simulink model "CognitiveOperator"  (R2017a)
settings: Solver=VariableStepAuto  StartTime=0.0  StopTime=81  RelTol=1e-3
values from neighbouring files (symbols this model uses):
  b = 0.1    [DCMotVal.mat]
  J = 0.01    [DCMotVal.mat]
  K = 0.01    [DCMotVal.mat]
  L = 0.5    [DCMotVal.mat]
  R = 1    [DCMotVal.mat]
libraries: simulink x1
settings Model: PauseTimes=1  Creator=Igor Khimchenko  LastModifiedBy=Igor Khimchenko

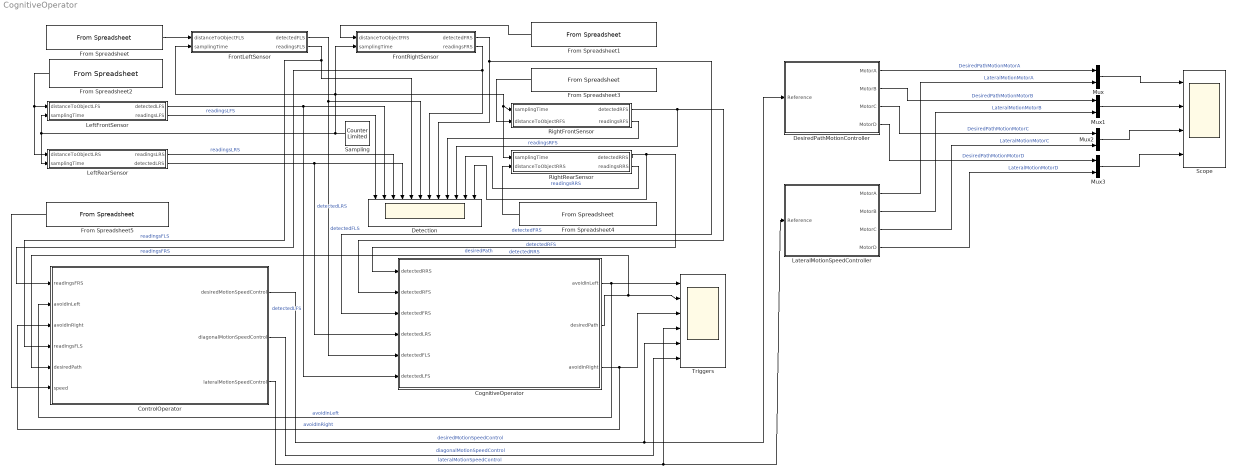
== system CognitiveOperator ==
  CognitiveOperator : Stateflow chart  TreatAsAtomicUnit=on
  ControlOperator : Stateflow chart  TreatAsAtomicUnit=on
  DesiredPathMotionController : Subsystem
  Detection : Scope  NumInputPorts=12
  From Spreadsheet : FromSpreadsheet  FileName=SensorReadings.xlsx  SheetName=Front left
  From Spreadsheet1 : FromSpreadsheet  FileName=SensorReadings.xlsx  SheetName=Front right
  From Spreadsheet2 : FromSpreadsheet  FileName=SensorReadings.xlsx  SheetName=Left
  From Spreadsheet3 : FromSpreadsheet  FileName=SensorReadings.xlsx  SheetName=Right front
  From Spreadsheet4 : FromSpreadsheet  FileName=SensorReadings.xlsx  SheetName=Right rear
  From Spreadsheet5 : FromSpreadsheet  FileName=SensorReadings.xlsx  SheetName=Speed
  FrontLeftSensor : Stateflow chart  TreatAsAtomicUnit=on
  FrontRightSensor : Stateflow chart  TreatAsAtomicUnit=on
  LateralMotionSpeedController : Subsystem
  LeftFrontSensor : Stateflow chart  TreatAsAtomicUnit=on
  LeftRearSensor : Stateflow chart  TreatAsAtomicUnit=on
  Mux{,1..3} (4 alike) : Mux  Inputs=2
  RightFrontSensor : Stateflow chart  TreatAsAtomicUnit=on
  RightRearSensor : Stateflow chart  TreatAsAtomicUnit=on
  Sampling : simulink/Sources/Counter Limited  uplimit=50  tsamp=0.001
  Scope : Scope  NumInputPorts=4
  Triggers : Scope  NumInputPorts=6
  wires:
  From Spreadsheet2/1 -> LeftRearSensor/1(distanceToObjectLRS), LeftFrontSensor/1(distanceToObjectLFS)
  Sampling/1 -> LeftRearSensor/2(samplingTime), LeftFrontSensor/2(samplingTime), FrontRightSensor/2(samplingTime), RightRearSensor/1(samplingTime), RightFrontSensor/1(samplingTime), FrontLeftSensor/2(samplingTime)
  LeftFrontSensor/2(readingsLFS) -> Detection/1  "readingsLFS"
  LeftFrontSensor/1(detectedLFS) -> CognitiveOperator/6(detectedLFS), Detection/2  "detectedLFS"
  LeftRearSensor/1(readingsLRS) -> Detection/3  "readingsLRS"
  LeftRearSensor/2(detectedLRS) -> CognitiveOperator/4(detectedLRS), Detection/4  "detectedLRS"
  FrontLeftSensor/2(readingsFLS) -> ControlOperator/4(readingsFLS), Detection/5  "readingsFLS"
  FrontLeftSensor/1(detectedFLS) -> CognitiveOperator/5(detectedFLS), Detection/6  "detectedFLS"
  FrontRightSensor/2(readingsFRS) -> ControlOperator/1(readingsFRS), Detection/7  "readingsFRS"
  FrontRightSensor/1(detectedFRS) -> CognitiveOperator/3(detectedFRS), Detection/8  "detectedFRS"
  RightFrontSensor/2(readingsRFS) -> Detection/9  "readingsRFS"
  RightFrontSensor/1(detectedRFS) -> Detection/10, CognitiveOperator/2(detectedRFS)  "detectedRFS"
  RightRearSensor/2(readingsRRS) -> Detection/11  "readingsRRS"
  RightRearSensor/1(detectedRRS) -> CognitiveOperator/1(detectedRRS), Detection/12  "detectedRRS"
  CognitiveOperator/1(avoidInLeft) -> ControlOperator/2(avoidInLeft), Triggers/1  "avoidInLeft"
  CognitiveOperator/2(desiredPath) -> ControlOperator/5(desiredPath), Triggers/2  "desiredPath"
  CognitiveOperator/3(avoidInRight) -> ControlOperator/3(avoidInRight), Triggers/3  "avoidInRight"
  From Spreadsheet3/1 -> RightFrontSensor/2(distanceToObjectRFS)
  From Spreadsheet4/1 -> RightRearSensor/2(distanceToObjectRRS)
  ControlOperator/1(desiredMotionSpeedControl) -> Triggers/5, DesiredPathMotionController/1(Reference)  "desiredMotionSpeedControl"
  ControlOperator/3(lateralMotionSpeedControl) -> Triggers/4, LateralMotionSpeedController/1(Reference)  "lateralMotionSpeedControl"
  From Spreadsheet5/1 -> ControlOperator/6(speed)
  From Spreadsheet/1 -> FrontLeftSensor/1(distanceToObjectFLS)
  From Spreadsheet1/1 -> FrontRightSensor/1(distanceToObjectFRS)
  ControlOperator/2(diagonalMotionSpeedControl) -> Triggers/6  "diagonalMotionSpeedControl"
  Mux/1 -> Scope/1
  Mux1/1 -> Scope/2
  Mux2/1 -> Scope/3
  Mux3/1 -> Scope/4
  DesiredPathMotionController/1(MotorA) -> Mux/1  "DesiredPathMotionMotorA"
  DesiredPathMotionController/2(MotorB) -> Mux1/1  "DesiredPathMotionMotorB"
  DesiredPathMotionController/3(MotorC) -> Mux2/1  "DesiredPathMotionMotorC"
  DesiredPathMotionController/4(MotorD) -> Mux3/1  "DesiredPathMotionMotorD"
  LateralMotionSpeedController/1(MotorA) -> Mux/2  "LateralMotionMotorA"
  LateralMotionSpeedController/2(MotorB) -> Mux1/2  "LateralMotionMotorB"
  LateralMotionSpeedController/3(MotorC) -> Mux2/2  "LateralMotionMotorC"
  LateralMotionSpeedController/4(MotorD) -> Mux3/2  "LateralMotionMotorD"

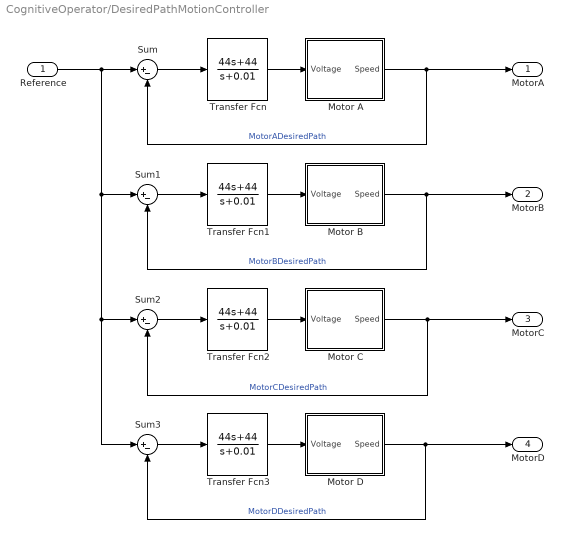
== system CognitiveOperator/DesiredPathMotionController ==
  Reference : Inport
  Motor A : Subsystem
  Motor B : Subsystem
  Motor C : Subsystem
  Motor D : Subsystem
  Sum{,1..3} (4 alike) : Sum  Inputs=|+-
  Transfer Fcn{,1..3} (4 alike) : TransferFcn  Numerator=[44 44]  Denominator=[1 0.01]
  MotorA : Outport
  MotorB : Outport  Port=2
  MotorC : Outport  Port=3
  MotorD : Outport  Port=4
  wires:
  Transfer Fcn/1 -> Motor A/1(Voltage)
  Sum2/1 -> Transfer Fcn2/1
  Transfer Fcn1/1 -> Motor B/1(Voltage)
  Sum1/1 -> Transfer Fcn1/1
  Motor D/1(Speed) -> MotorD/1, Sum3/2  "MotorDDesiredPath"
  Sum3/1 -> Transfer Fcn3/1
  Motor A/1(Speed) -> MotorA/1, Sum/2  "MotorADesiredPath"
  Motor C/1(Speed) -> MotorC/1, Sum2/2  "MotorCDesiredPath"
  Sum/1 -> Transfer Fcn/1
  Transfer Fcn3/1 -> Motor D/1(Voltage)
  Reference/1 -> Sum3/1, Sum2/1, Sum1/1, Sum/1
  Motor B/1(Speed) -> MotorB/1, Sum1/2  "MotorBDesiredPath"
  Transfer Fcn2/1 -> Motor C/1(Voltage)

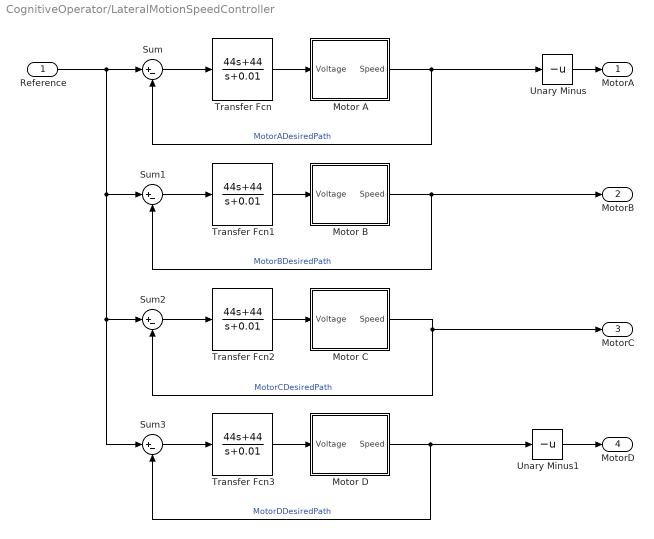
== system CognitiveOperator/LateralMotionSpeedController ==
  Reference : Inport
  Motor A : Subsystem
  Motor B : Subsystem
  Motor C : Subsystem
  Motor D : Subsystem
  Sum{,1..3} (4 alike) : Sum  Inputs=|+-
  Transfer Fcn{,1..3} (4 alike) : TransferFcn  Numerator=[44 44]  Denominator=[1 0.01]
  Unary Minus : UnaryMinus
  Unary Minus1 : UnaryMinus
  MotorA : Outport
  MotorB : Outport  Port=2
  MotorC : Outport  Port=3
  MotorD : Outport  Port=4
  wires:
  Sum/1 -> Transfer Fcn/1
  Transfer Fcn/1 -> Motor A/1(Voltage)
  Sum2/1 -> Transfer Fcn2/1
  Sum3/1 -> Transfer Fcn3/1
  Motor C/1(Speed) -> MotorC/1, Sum2/2  "MotorCDesiredPath"
  Sum1/1 -> Transfer Fcn1/1
  Transfer Fcn3/1 -> Motor D/1(Voltage)
  Reference/1 -> Sum3/1, Sum2/1, Sum1/1, Sum/1
  Transfer Fcn1/1 -> Motor B/1(Voltage)
  Transfer Fcn2/1 -> Motor C/1(Voltage)
  Motor B/1(Speed) -> MotorB/1, Sum1/2  "MotorBDesiredPath"
  Motor D/1(Speed) -> Unary Minus1/1, Sum3/2  "MotorDDesiredPath"
  Motor A/1(Speed) -> Unary Minus/1, Sum/2  "MotorADesiredPath"
  Unary Minus/1 -> MotorA/1
  Unary Minus1/1 -> MotorD/1

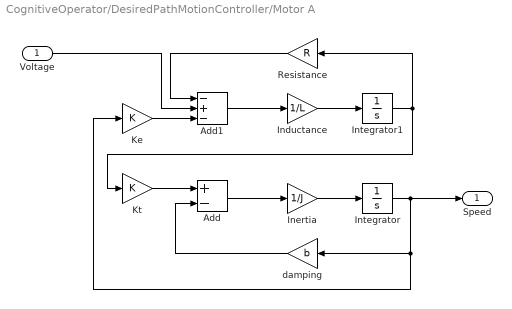
== system CognitiveOperator/DesiredPathMotionController/Motor A ==
  Voltage : Inport
  Add : Sum  Inputs=+-
  Add1 : Sum  Inputs=-+-
  Inductance : Gain  Gain=1/L
  Inertia : Gain  Gain=1/J
  Integrator : Integrator
  Integrator1 : Integrator
  Ke : Gain  Gain=K
  Kt : Gain  Gain=K
  Resistance : Gain  Gain=R
  damping : Gain  Gain=b
  Speed : Outport
  wires:
  Resistance/1 -> Add1/1
  Inductance/1 -> Integrator1/1
  Kt/1 -> Add/1
  Ke/1 -> Add1/3
  Inertia/1 -> Integrator/1
  Add1/1 -> Inductance/1
  Integrator/1 -> Ke/1, damping/1, Speed/1
  damping/1 -> Add/2
  Voltage/1 -> Add1/2
  Integrator1/1 -> Resistance/1, Kt/1
  Add/1 -> Inertia/1

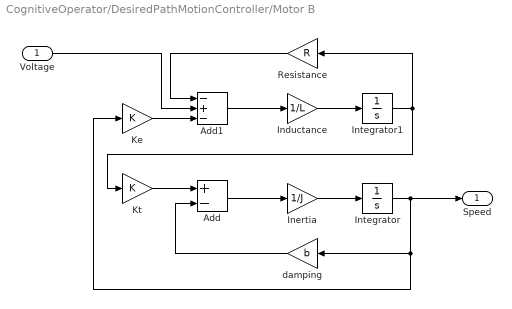
== system CognitiveOperator/DesiredPathMotionController/Motor B ==
  Voltage : Inport
  Add : Sum  Inputs=+-
  Add1 : Sum  Inputs=-+-
  Inductance : Gain  Gain=1/L
  Inertia : Gain  Gain=1/J
  Integrator : Integrator
  Integrator1 : Integrator
  Ke : Gain  Gain=K
  Kt : Gain  Gain=K
  Resistance : Gain  Gain=R
  damping : Gain  Gain=b
  Speed : Outport
  wires:
  Resistance/1 -> Add1/1
  Inductance/1 -> Integrator1/1
  Kt/1 -> Add/1
  Ke/1 -> Add1/3
  Inertia/1 -> Integrator/1
  Add1/1 -> Inductance/1
  Integrator/1 -> Ke/1, damping/1, Speed/1
  damping/1 -> Add/2
  Voltage/1 -> Add1/2
  Integrator1/1 -> Resistance/1, Kt/1
  Add/1 -> Inertia/1

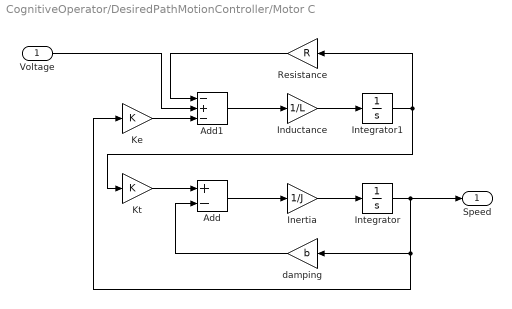
== system CognitiveOperator/DesiredPathMotionController/Motor C ==
  Voltage : Inport
  Add : Sum  Inputs=+-
  Add1 : Sum  Inputs=-+-
  Inductance : Gain  Gain=1/L
  Inertia : Gain  Gain=1/J
  Integrator : Integrator
  Integrator1 : Integrator
  Ke : Gain  Gain=K
  Kt : Gain  Gain=K
  Resistance : Gain  Gain=R
  damping : Gain  Gain=b
  Speed : Outport
  wires:
  Resistance/1 -> Add1/1
  Inductance/1 -> Integrator1/1
  Kt/1 -> Add/1
  Ke/1 -> Add1/3
  Inertia/1 -> Integrator/1
  Add1/1 -> Inductance/1
  Integrator/1 -> Ke/1, damping/1, Speed/1
  damping/1 -> Add/2
  Voltage/1 -> Add1/2
  Integrator1/1 -> Resistance/1, Kt/1
  Add/1 -> Inertia/1

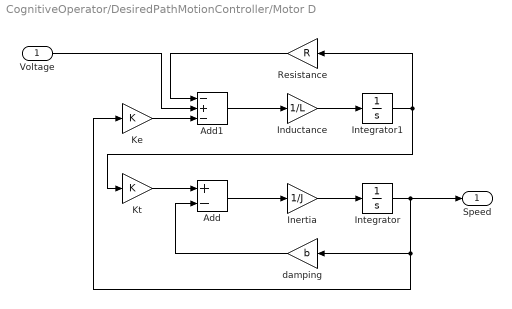
== system CognitiveOperator/DesiredPathMotionController/Motor D ==
  Voltage : Inport
  Add : Sum  Inputs=+-
  Add1 : Sum  Inputs=-+-
  Inductance : Gain  Gain=1/L
  Inertia : Gain  Gain=1/J
  Integrator : Integrator
  Integrator1 : Integrator
  Ke : Gain  Gain=K
  Kt : Gain  Gain=K
  Resistance : Gain  Gain=R
  damping : Gain  Gain=b
  Speed : Outport
  wires:
  Resistance/1 -> Add1/1
  Inductance/1 -> Integrator1/1
  Kt/1 -> Add/1
  Ke/1 -> Add1/3
  Inertia/1 -> Integrator/1
  Add1/1 -> Inductance/1
  Integrator/1 -> Ke/1, damping/1, Speed/1
  damping/1 -> Add/2
  Voltage/1 -> Add1/2
  Integrator1/1 -> Resistance/1, Kt/1
  Add/1 -> Inertia/1

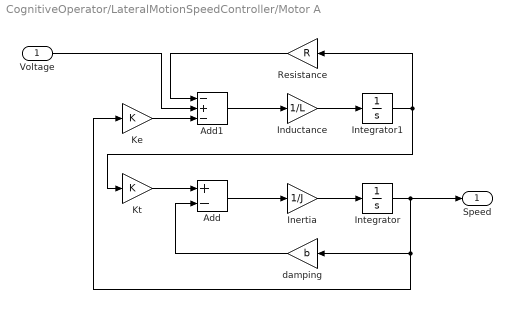
== system CognitiveOperator/LateralMotionSpeedController/Motor A ==
  Voltage : Inport
  Add : Sum  Inputs=+-
  Add1 : Sum  Inputs=-+-
  Inductance : Gain  Gain=1/L
  Inertia : Gain  Gain=1/J
  Integrator : Integrator
  Integrator1 : Integrator
  Ke : Gain  Gain=K
  Kt : Gain  Gain=K
  Resistance : Gain  Gain=R
  damping : Gain  Gain=b
  Speed : Outport
  wires:
  Resistance/1 -> Add1/1
  Inductance/1 -> Integrator1/1
  Kt/1 -> Add/1
  Ke/1 -> Add1/3
  Inertia/1 -> Integrator/1
  Add1/1 -> Inductance/1
  Integrator/1 -> Ke/1, damping/1, Speed/1
  damping/1 -> Add/2
  Voltage/1 -> Add1/2
  Integrator1/1 -> Resistance/1, Kt/1
  Add/1 -> Inertia/1

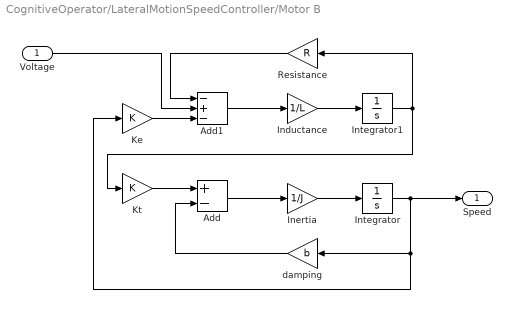
== system CognitiveOperator/LateralMotionSpeedController/Motor B ==
  Voltage : Inport
  Add : Sum  Inputs=+-
  Add1 : Sum  Inputs=-+-
  Inductance : Gain  Gain=1/L
  Inertia : Gain  Gain=1/J
  Integrator : Integrator
  Integrator1 : Integrator
  Ke : Gain  Gain=K
  Kt : Gain  Gain=K
  Resistance : Gain  Gain=R
  damping : Gain  Gain=b
  Speed : Outport
  wires:
  Resistance/1 -> Add1/1
  Inductance/1 -> Integrator1/1
  Kt/1 -> Add/1
  Ke/1 -> Add1/3
  Inertia/1 -> Integrator/1
  Add1/1 -> Inductance/1
  Integrator/1 -> Ke/1, damping/1, Speed/1
  damping/1 -> Add/2
  Voltage/1 -> Add1/2
  Integrator1/1 -> Resistance/1, Kt/1
  Add/1 -> Inertia/1

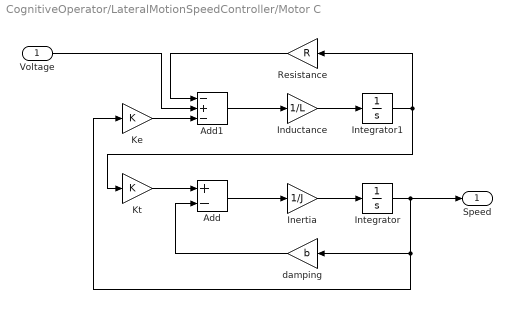
== system CognitiveOperator/LateralMotionSpeedController/Motor C ==
  Voltage : Inport
  Add : Sum  Inputs=+-
  Add1 : Sum  Inputs=-+-
  Inductance : Gain  Gain=1/L
  Inertia : Gain  Gain=1/J
  Integrator : Integrator
  Integrator1 : Integrator
  Ke : Gain  Gain=K
  Kt : Gain  Gain=K
  Resistance : Gain  Gain=R
  damping : Gain  Gain=b
  Speed : Outport
  wires:
  Resistance/1 -> Add1/1
  Inductance/1 -> Integrator1/1
  Kt/1 -> Add/1
  Ke/1 -> Add1/3
  Inertia/1 -> Integrator/1
  Add1/1 -> Inductance/1
  Integrator/1 -> Ke/1, damping/1, Speed/1
  damping/1 -> Add/2
  Voltage/1 -> Add1/2
  Integrator1/1 -> Resistance/1, Kt/1
  Add/1 -> Inertia/1

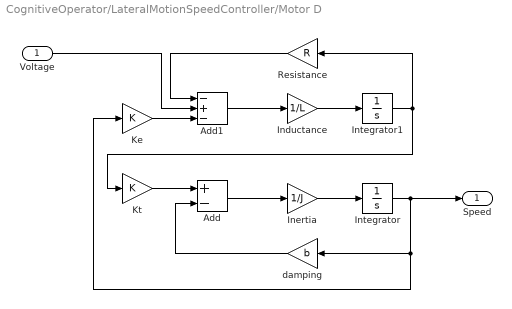
== system CognitiveOperator/LateralMotionSpeedController/Motor D ==
  Voltage : Inport
  Add : Sum  Inputs=+-
  Add1 : Sum  Inputs=-+-
  Inductance : Gain  Gain=1/L
  Inertia : Gain  Gain=1/J
  Integrator : Integrator
  Integrator1 : Integrator
  Ke : Gain  Gain=K
  Kt : Gain  Gain=K
  Resistance : Gain  Gain=R
  damping : Gain  Gain=b
  Speed : Outport
  wires:
  Resistance/1 -> Add1/1
  Inductance/1 -> Integrator1/1
  Kt/1 -> Add/1
  Ke/1 -> Add1/3
  Inertia/1 -> Integrator/1
  Add1/1 -> Inductance/1
  Integrator/1 -> Ke/1, damping/1, Speed/1
  damping/1 -> Add/2
  Voltage/1 -> Add1/2
  Integrator1/1 -> Resistance/1, Kt/1
  Add/1 -> Inertia/1

== stateflow chart CognitiveOperator/LeftFrontSensor ==
  state LFSEnvironmentSampling
    entry: detectedLFS = 0
    readingsLFS = distanceToObjectLFS
  state LFSObstacleDetected
    entry: detectedLFS = 1
    readingsLFS = distanceToObjectLFS
  (default) -> LFSEnvironmentSampling
  LFSEnvironmentSampling -> LFSEnvironmentSampling [order 2] : [samplingTime == 50]
  LFSEnvironmentSampling -> LFSObstacleDetected [order 1] : [distanceToObjectLFS <= 1]
  LFSObstacleDetected -> LFSEnvironmentSampling [order 1] : [not(distanceToObjectLFS <= 1)]
  LFSObstacleDetected -> LFSObstacleDetected [order 2] : [samplingTime == 50]
  data: distanceToObjectLFS input; samplingTime input; detectedLFS output; readingsLFS output

== stateflow chart CognitiveOperator/LeftRearSensor ==
  state LRSEnvironmentSampling
    entry: detectedLRS = 0
    readingsLRS = distanceToObjectLRS
  state LRSObstacleDetected
    entry: detectedLRS = 1
    readingsLRS = distanceToObjectLRS
  (default) -> LRSEnvironmentSampling
  LRSEnvironmentSampling -> LRSEnvironmentSampling [order 2] : [samplingTime == 50]
  LRSEnvironmentSampling -> LRSObstacleDetected [order 1] : [distanceToObjectLRS <= 1]
  LRSObstacleDetected -> LRSEnvironmentSampling [order 1] : [not(distanceToObjectLRS <= 1)]
  LRSObstacleDetected -> LRSObstacleDetected [order 2] : [samplingTime == 50]
  data: distanceToObjectLRS input; samplingTime input; readingsLRS output; detectedLRS output

== stateflow chart CognitiveOperator/CognitiveOperator ==
  state DesiredPathTrigger
    entry: avoidInLeft = 0
    avoidInRight = 0
    desiredPath = 1
  state AvoidInLeftTrigger
    entry: avoidInLeft = 1
    avoidInRight = 0
    desiredPath = 0
  state AvoidInRightTrigger
    entry: avoidInLeft = 0
    avoidInRight = 1
    desiredPath = 0
  (default) -> DesiredPathTrigger
  DesiredPathTrigger -> AvoidInLeftTrigger [order 2] : [not(detectedLRS && detectedLFS) && (detectedFLS && detectedFRS) && (detectedRFS && detectedRRS)]
  DesiredPathTrigger -> AvoidInRightTrigger [order 1] : [not(detectedRRS && detectedRFS) && (detectedFLS && detectedFRS) && (detectedLFS && detectedLRS)]
  AvoidInLeftTrigger -> DesiredPathTrigger : [not(detectedFLS) && not(detectedFRS)]
  AvoidInRightTrigger -> DesiredPathTrigger : [not(detectedFLS) && not(detectedFRS)]
  data: detectedRRS input; detectedRFS input; detectedFRS input; detectedLRS input; detectedFLS input; detectedLFS input; avoidInLeft output; desiredPath output; avoidInRight output

== stateflow chart CognitiveOperator/FrontLeftSensor ==
  state FLSEnvironmentSampling
    entry: detectedFLS = 0
    readingsFLS = distanceToObjectFLS
  state FLSObstacleDetected
    entry: detectedFLS = 1
    readingsFLS = distanceToObjectFLS
  (default) -> FLSEnvironmentSampling
  FLSEnvironmentSampling -> FLSEnvironmentSampling [order 2] : [samplingTime == 50]
  FLSEnvironmentSampling -> FLSObstacleDetected [order 1] : [distanceToObjectFLS <= 1]
  FLSObstacleDetected -> FLSEnvironmentSampling [order 1] : [not(distanceToObjectFLS <= 1)]
  FLSObstacleDetected -> FLSObstacleDetected [order 2] : [samplingTime == 50]
  data: distanceToObjectFLS input; samplingTime input; detectedFLS output; readingsFLS output

== stateflow chart CognitiveOperator/FrontRightSensor ==
  state FRSEnvironmentSampling
    entry: detectedFRS = 0
    readingsFRS = distanceToObjectFRS
  state FRSObstacleDetected
    entry: detectedFRS = 1
    readingsFRS = distanceToObjectFRS
  (default) -> FRSEnvironmentSampling
  FRSEnvironmentSampling -> FRSEnvironmentSampling [order 2] : [samplingTime == 50]
  FRSEnvironmentSampling -> FRSObstacleDetected [order 1] : [distanceToObjectFRS <= 1]
  FRSObstacleDetected -> FRSEnvironmentSampling [order 1] : [not(distanceToObjectFRS <= 1)]
  FRSObstacleDetected -> FRSObstacleDetected [order 2] : [samplingTime == 50]
  data: distanceToObjectFRS input; samplingTime input; detectedFRS output; readingsFRS output

== stateflow chart CognitiveOperator/RightFrontSensor ==
  state RFSEnvironmentSampling
    entry: detectedRFS = 0
    readingsRFS = distanceToObjectRFS
  state RFSObstacleDetected
    entry: detectedRFS = 1
    readingsRFS = distanceToObjectRFS
  (default) -> RFSEnvironmentSampling
  RFSEnvironmentSampling -> RFSEnvironmentSampling [order 2] : [samplingTime == 50]
  RFSEnvironmentSampling -> RFSObstacleDetected [order 1] : [distanceToObjectRFS <= 1]
  RFSObstacleDetected -> RFSEnvironmentSampling [order 1] : [not(distanceToObjectRFS <= 1)]
  RFSObstacleDetected -> RFSObstacleDetected [order 2] : [samplingTime == 50]
  data: samplingTime input; distanceToObjectRFS input; detectedRFS output; readingsRFS output

== stateflow chart CognitiveOperator/RightRearSensor ==
  state RRSEnvironmentSampling
    entry: detectedRRS = 0
    readingsRRS = distanceToObjectRRS
  state RRSObstacleDetected
    entry: detectedRRS = 1
    readingsRRS = distanceToObjectRRS
  (default) -> RRSEnvironmentSampling
  RRSEnvironmentSampling -> RRSEnvironmentSampling [order 2] : [samplingTime == 50]
  RRSEnvironmentSampling -> RRSObstacleDetected [order 1] : [distanceToObjectRRS <= 1]
  RRSObstacleDetected -> RRSEnvironmentSampling [order 1] : [not(distanceToObjectRRS <= 1)]
  RRSObstacleDetected -> RRSObstacleDetected [order 2] : [samplingTime == 50]
  data: samplingTime input; distanceToObjectRRS input; detectedRRS output; readingsRRS output

== stateflow chart CognitiveOperator/ControlOperator ==
  state LateralMotionSpeedControl
    entry: lateralMotionSpeedControl = 1
    desiredMotionSpeedControl = 0
    diagonalMotionSpeedControl = 0
  state DesiredMotionSpeedControl
    entry: lateralMotionSpeedControl = 0
    desiredMotionSpeedControl = 1
    diagonalMotionSpeedControl = 0
  state DiagonalMotionSpeedControl
    entry: lateralMotionSpeedControl = 0
    desiredMotionSpeedControl = 0
    diagonalMotionSpeedControl = 1
  (default) -> DesiredMotionSpeedControl
  DesiredMotionSpeedControl -> LateralMotionSpeedControl [order 1] : [(avoidInLeft | avoidInRight) & (readingsFLS < 0.3 & readingsFRS < 0.3) & speed == 0]
  DesiredMotionSpeedControl -> DiagonalMotionSpeedControl [order 2] : [(avoidInLeft | avoidInRight) & (readingsFLS < 0.2 | readingsFRS <  0.2 ) & not(readingsFLS <  0.2 & readingsFRS < 0.2) & speed == 0]
  DiagonalMotionSpeedControl -> DesiredMotionSpeedControl : [desiredPath & speed == 0]
  LateralMotionSpeedControl -> DesiredMotionSpeedControl : [desiredPath & speed == 0]
  data: readingsFRS input; avoidInLeft input; avoidInRight input; readingsFLS input; desiredPath input; speed input; desiredMotionSpeedControl output; diagonalMotionSpeedControl output; lateralMotionSpeedControl output
